simulink model "SimulinkAnalysisofCheetahTail"  (R2022a)
settings: Solver=ode4  StartTime=0.0  StopTime=1.5  FixedStep=0.001  RelTol=1e-3
undefined symbols (not defined in the file): B_cg_H, B_con_H, B_con_L, bar_len, cd_table, Cf, cl_table, g, gear_ratio, int_point_bar, int_point_tail, ITail, M_add, M_cg_H, M_cg_L, M_cg_W, Mb, Mm, Mt, psi3, rho, T_cg_H, T_fur_gap, T_length, T_width_major, T_width_minor, th2_initial, torque_constant, uncertainty_Forces, uncertainty_Position, Vf, windspeed
(part 17 of 21)

== matlab function SimulinkAnalysisofCheetahTail/Model/Forces/MATLAB Function1 ==
  data: int_point_tail input; A_output output; bar_len parameter; T_length parameter; T_width_major parameter
function A_output = fcn(int_point_tail, bar_len, T_length, T_width_major)

A_output = (T_length + bar_len-int_point_tail)/5*T_width_major;

== matlab function SimulinkAnalysisofCheetahTail/Model/Forces/CD_CL_tail_1/v_tail_1 ==
  data: v_tail_1_speed output; int_point_tail input; q input; dq input; B_con_H parameter; psi3 parameter; windspeed parameter; B_con_L parameter; M_cg_H parameter; M_cg_L parameter; M_cg_W parameter; T_fur_gap parameter; T_length parameter; bar_len parameter
function v_tail_1_speed = v_tail_1(int_point_tail,q,dq, B_con_H, psi3, windspeed, B_con_L, M_cg_H, M_cg_L, M_cg_W, T_fur_gap, T_length, bar_len)
%#codegen
[x,y,z,phi1,th1,psi1,phi2,th2] = deal(q(1),q(2),q(3),q(4),q(5),q(6),q(7),q(8));
[dx,dy,dz,dphi1,dth1,dpsi1,dphi2,dth2] = deal(dq(1),dq(2),dq(3),dq(4),dq(5),dq(6),dq(7),dq(8));
%    This function was generated by the Symbolic Math Toolbox version 9.0.
%    09-Feb-2022 11:07:13

t2 = cos(phi1);
t3 = cos(phi2);
t4 = cos(psi1);
t5 = cos(psi3);
t6 = cos(th1);
t7 = cos(th2);
t8 = sin(phi1);
t9 = sin(phi2);
t10 = sin(psi1);
t11 = sin(psi3);
t12 = sin(th1);
t13 = sin(th2);
t14 = M_cg_L+x;
t15 = M_cg_W+y;
t16 = M_cg_H+z;
t35 = T_length./1.0e+1;
t36 = bar_len./1.0e+1;
t37 = int_point_tail./1.0e+1;
t17 = B_con_L.*t6;
t18 = B_con_L.*t12;
t19 = t2.*t4;
t20 = t6.*t7;
t21 = t2.*t10;
t22 = t4.*t8;
t23 = t7.*t12;
t24 = t8.*t10;
t25 = t12.*t13;
t26 = B_con_H.*t2.*t6;
t28 = t6.*t14;
t29 = B_con_H.*t2.*t12;
t30 = B_con_H.*t6.*t8;
t33 = t12.*t14;
t40 = t6.*t9.*t13;
t42 = t6.*t10.*t13;
t44 = t8.*t9.*t12;
t47 = -t37;
t48 = t2.*t3.*t6;
t51 = t2.*t6.*t9;
t52 = t3.*t6.*t8;
t54 = t2.*t6.*t13;
t55 = t3.*t6.*t13;
t57 = t4.*t6.*t13;
t60 = t3.*t8.*t12;
t61 = t6.*t8.*t9;
t66 = t2.*t6.*t15;
t68 = t2.*t6.*t16;
t71 = t6.*t8.*t15;
t72 = t2.*t12.*t16;
t73 = t6.*t8.*t16;
t75 = t8.*t12.*t15;
t27 = t4.*t17;
t31 = t4.*t18;
t32 = t10.*t17;
t34 = t10.*t18;
t38 = t2.*t25;
t39 = t3.*t25;
t41 = t9.*t23;
t43 = t10.*t23;
t45 = t12.*t24;
t46 = t9.*t25;
t49 = t2.*t20;
t50 = t4.*t20;
t53 = t12.*t19;
t56 = t3.*t23;
t58 = t4.*t23;
t59 = t10.*t20;
t62 = t12.*t21;
t63 = t12.*t22;
t64 = B_con_H.*t6.*t19;
t65 = t4.*t28;
t67 = B_con_H.*t6.*t21;
t69 = t4.*t33;
t70 = t10.*t28;
t74 = t10.*t33;
t76 = -t29;
t77 = -t30;
t79 = -t44;
t84 = t3.*t6.*t22;
t85 = t13.*t48;
t88 = t3.*t8.*t20;
t89 = t6.*t13.*t19;
t90 = t4.*t55;
t93 = t3.*t6.*t24;
t94 = t6.*t9.*t22;
t95 = t2.*t40;
t97 = t8.*t9.*t20;
t98 = t6.*t13.*t21;
t100 = t3.*t42;
t101 = t4.*t40;
t103 = t6.*t9.*t24;
t107 = t10.*t40;
t109 = -t57;
t112 = t6.*t16.*t19;
t113 = t6.*t15.*t22;
t114 = t6.*t16.*t21;
t115 = t6.*t15.*t24;
t116 = -t66;
t117 = -t71;
t118 = -t72;
t119 = -t73;
t120 = t3.*t19.*t20;
t121 = t3.*t20.*t21;
t122 = t9.*t19.*t20;
t123 = t9.*t20.*t21;
t133 = t23+t54;
t194 = t35+t36+t47;
t78 = -t38;
t80 = -t45;
t81 = -t46;
t82 = t3.*t49;
t83 = t3.*t50;
t86 = t2.*t56;
t87 = t9.*t49;
t91 = t3.*t59;
t92 = t9.*t50;
t96 = t2.*t41;
t99 = t4.*t39;
t102 = t9.*t59;
t104 = -t49;
t105 = t10.*t39;
t106 = t4.*t46;
t108 = -t53;
t110 = -t59;
t111 = t10.*t46;
t125 = -t90;
t127 = -t97;
t131 = -t113;
t132 = -t115;
t134 = t21+t63;
t135 = t22+t62;
t136 = -t120;
t137 = -t121;
t144 = t5.*t133;
t148 = t11.*t133;
t152 = t51+t88;
t156 = t56+t85;
t157 = t58+t89;
t158 = t41+t95;
t159 = t43+t98;
t124 = -t82;
t126 = -t91;
t128 = -t102;
t129 = t4.*t81;
t130 = t10.*t81;
t138 = B_con_H.*t134;
t139 = B_con_H.*t135;
t140 = t20+t78;
t141 = t25+t104;
t142 = t19+t80;
t143 = t24+t108;
t145 = t3.*t134;
t146 = t3.*t135;
t147 = t7.*t135;
t149 = t9.*t134;
t150 = t9.*t135;
t151 = t13.*t135;
t160 = t15.*t134;
t161 = t15.*t135;
t162 = t16.*t134;
t163 = t16.*t135;
t173 = -t148;
t177 = t48+t127;
t178 = T_fur_gap.*t152;
t179 = T_fur_gap.*t156;
t180 = int_point_tail.*t152;
t181 = int_point_tail.*t156;
t202 = t40+t60+t96;
t205 = t55+t79+t86;
t206 = t52+t81+t87;
t229 = t94+t99+t136;
t231 = t103+t105+t137;
t239 = t152.*t194;
t240 = t156.*t194;
t153 = B_con_H.*t142;
t154 = B_con_H.*t143;
t155 = -t139;
t164 = t7.*t145;
t165 = t7.*t146;
t166 = t13.*t146;
t167 = t7.*t149;
t168 = t9.*t147;
t169 = t13.*t150;
t170 = t3.*t142;
t171 = t3.*t143;
t172 = t7.*t143;
t174 = t9.*t142;
t175 = t9.*t143;
t176 = t13.*t143;
t182 = t15.*t142;
t183 = t15.*t143;
t184 = -t161;
t185 = t16.*t142;
t186 = t16.*t143;
t187 = -t163;
t201 = t42+t147;
t203 = t110+t151;
t204 = t39+t61+t124;
t209 = T_fur_gap.*t205;
t210 = T_fur_gap.*t206;
t212 = int_point_tail.*t205;
t213 = int_point_tail.*t206;
t216 = -t5.*(t59-t151);
t218 = -t11.*(t59-t151);
t219 = t5.*t206;
t220 = t11.*t206;
t230 = t84+t122+t129;
t232 = t93+t123+t130;
t233 = T_fur_gap.*t229;
t234 = int_point_tail.*t229;
t235 = T_fur_gap.*t231;
t236 = int_point_tail.*t231;
t250 = t194.*t205;
t251 = t194.*t206;
t272 = t194.*t229;
t275 = t194.*t231;
t283 = t179+t181+t240;
t289 = t77+t116+t119+t178+t180+t239;
t188 = t7.*t170;
t189 = t7.*t171;
t190 = -t164;
t191 = t13.*t171;
t192 = t7.*t174;
t193 = t9.*t172;
t195 = t13.*t175;
t196 = -t170;
t197 = -t182;
t198 = -t183;
t207 = t50+t176;
t208 = T_fur_gap.*t204;
t211 = int_point_tail.*t204;
t214 = t109+t172;
t222 = t126+t166;
t224 = t128+t169;
t226 = -T_fur_gap.*(t91-t166);
t228 = -int_point_tail.*(t91-t166);
t238 = t167+t171;
t244 = -T_fur_gap.*(t164-t175);
t246 = -int_point_tail.*(t164-t175);
t247 = t144+t220;
t248 = t100+t165+t174;
t249 = t194.*t204;
t255 = t173+t219;
t268 = -t194.*(t91-t166);
t277 = -t194.*(t164-t175);
t288 = t210+t213+t251;
t293 = t17+t28+t75+t76+t118+t209+t212+t250;
t294 = t34+t67+t74+t114+t132+t235+t236+t275;
t295 = t31+t64+t69+t112+t131+t233+t234+t272;
t199 = -t188;
t200 = -t193;
t215 = t5.*t207;
t217 = t11.*t207;
t221 = t83+t191;
t223 = t92+t195;
t237 = t146+t192;
t242 = t175+t190;
t252 = T_fur_gap.*t248;
t253 = int_point_tail.*t248;
t254 = t125+t149+t189;
t257 = t107+t168+t196;
t278 = t194.*t248;
t291 = t226+t228+t268;
t292 = t18+t26+t33+t68+t117+t208+t211+t249;
t298 = t138+t162+t198+t244+t246+t277;
t225 = T_fur_gap.*t221;
t227 = int_point_tail.*t221;
t241 = t150+t199;
t256 = t101+t145+t200;
t258 = T_fur_gap.*t254;
t260 = int_point_tail.*t254;
t261 = T_fur_gap.*t257;
t263 = int_point_tail.*t257;
t265 = t194.*t221;
t266 = t5.*t257;
t269 = t11.*t257;
t279 = t194.*t254;
t281 = t194.*t257;
t300 = t32+t70+t155+t187+t197+t252+t253+t278;
t243 = T_fur_gap.*t241;
t245 = int_point_tail.*t241;
t259 = T_fur_gap.*t256;
t262 = int_point_tail.*t256;
t264 = t5.*t256;
t267 = t11.*t256;
t270 = -t258;
t271 = -t260;
t273 = -t266;
t276 = t194.*t241;
t280 = t194.*t256;
t282 = -t279;
t285 = t216+t269;
t290 = t225+t227+t265;
t297 = t261+t263+t281;
t274 = -t267;
t284 = t217+t264;
t287 = t218+t273;
t296 = t259+t262+t280;
t299 = t153+t184+t185+t243+t245+t276;
t301 = t27+t65+t154+t160+t186+t270+t271+t282;
t286 = t215+t274;
et1 = dphi1.*(t204.*(t30+t66+t73-t178-t180-t239)-t152.*t292+t241.*t300+t248.*t299+t301.*(t164-t175)-t254.*(-t138-t162+t183+T_fur_gap.*(t164-t175)+int_point_tail.*(t164-t175)+t194.*(t164-t175)))-dth2.*(t156.*t292+t204.*t283+t221.*t301-t254.*t290+t248.*(T_fur_gap.*(t91-t166)+int_point_tail.*(t91-t166)+t194.*(t91-t166))+t300.*(t91-t166))+dy.*(t134.*t254+t142.*t248+t6.*t8.*t204)+dz.*(t135.*t248+t143.*t254-t2.*t6.*t204)-dphi2.*(t204.*t288+t206.*t292-t248.*t297+t254.*t296-t256.*t301-t257.*t300);
et2 = -dth1.*(t204.*t293+t205.*t292-t229.*t301-t231.*t300-t248.*t294+t254.*t295)-dx.*(t12.*t204-t4.*t6.*t254+t6.*t10.*t248)+t5.*t248.*windspeed-t11.*t254.*windspeed;
et3 = dphi2.*(t297.*(t269-t5.*(t59-t151))+t247.*t288-t286.*t296-t11.*t204.*t292-t11.*t248.*t300+t11.*t254.*t301)+dth1.*(t294.*(t269-t5.*(t59-t151))+t247.*t293-t286.*t295+t292.*(t5.*t140-t11.*t202)-t301.*(t5.*t157+t11.*t230)-t300.*(t5.*t159+t11.*t232))+dy.*(t142.*(t269-t5.*(t59-t151))+t134.*t286-t6.*t8.*t247)+dz.*(t135.*(t269-t5.*(t59-t151))+t143.*t286+t2.*t6.*t247);
et4 = -dth2.*(-t247.*t283-t286.*t290+(t269-t5.*(t59-t151)).*(T_fur_gap.*(t91-t166)+int_point_tail.*(t91-t166)+t194.*(t91-t166))+t292.*(t5.*t141+t11.*t158)+t301.*(t11.*t223+t5.*(t57-t172))+t300.*(t5.*t201+t11.*(t102-t169)))+dx.*(t12.*t247-t6.*t10.*(t269-t5.*(t59-t151))+t4.*t6.*t286);
et5 = -dphi1.*(t247.*(t30+t66+t73-t178-t180-t239)-t299.*(t269-t5.*(t59-t151))-t301.*(t11.*t238+t5.*t13.*t134)+t300.*(t11.*t237+t5.*t13.*t142)+t286.*(-t138-t162+t183+T_fur_gap.*(t164-t175)+int_point_tail.*(t164-t175)+t194.*(t164-t175))-t292.*(t11.*t177-t5.*t6.*t8.*t13))+t5.*windspeed.*(t269-t5.*(t59-t151))-t11.*t286.*windspeed;
et6 = -dphi1.*(t299.*(t266+t11.*(t59-t151))+t301.*(t5.*t238-t11.*t13.*t134)-t300.*(t5.*t237-t11.*t13.*t142)+(t148-t219).*(t30+t66+t73-t178-t180-t239)+t284.*(-t138-t162+t183+T_fur_gap.*(t164-t175)+int_point_tail.*(t164-t175)+t194.*(t164-t175))+t292.*(t5.*t177+t6.*t8.*t11.*t13))-dphi2.*(t297.*(t266+t11.*(t59-t151))+t284.*t296-t288.*(t148-t219)-t5.*t204.*t292-t5.*t248.*t300+t5.*t254.*t301);
et7 = -dth1.*(t294.*(t266+t11.*(t59-t151))+t284.*t295-t293.*(t148-t219)-t292.*(t11.*t140+t5.*t202)+t301.*(t11.*t157-t5.*t230)+t300.*(t11.*t159-t5.*t232))-dy.*(t142.*(t266+t11.*(t59-t151))-t134.*t284+t6.*t8.*(t148-t219))+dz.*(-t135.*(t266+t11.*(t59-t151))+t143.*t284+t2.*t6.*(t148-t219));
et8 = dth2.*(t284.*t290+(t266+t11.*(t59-t151)).*(T_fur_gap.*(t91-t166)+int_point_tail.*(t91-t166)+t194.*(t91-t166))+t283.*(t148-t219)-t292.*(t11.*t141-t5.*t158)+t301.*(t5.*t223-t11.*(t57-t172))-t300.*(t11.*t201-t5.*(t102-t169)))+dx.*(t12.*(t148-t219)+t6.*t10.*(t266+t11.*(t59-t151))+t4.*t6.*t284)-t5.*windspeed.*(t266+t11.*(t59-t151))-t11.*t284.*windspeed;
v_tail_1_speed = sqrt(abs(et3+et4+et5).^2+abs(et6+et7+et8).^2+abs(et1+et2).^2);

== matlab function SimulinkAnalysisofCheetahTail/Model/Forces/CD_CL_tail_1/aoa_tail_1 ==
  data: int_point_tail input; q input; dq input; aoa_tail_1 output; psi3 parameter; windspeed parameter; B_con_H parameter; B_con_L parameter; M_cg_H parameter; M_cg_L parameter; M_cg_W parameter; T_fur_gap parameter; T_length parameter; bar_len parameter
function aoa_tail_1 = aoa_tail_1(int_point_tail,q,dq, psi3, windspeed, B_con_H, B_con_L, M_cg_H, M_cg_L, M_cg_W, T_fur_gap, T_length, bar_len)
%#codegen
[x,y,z,phi1,th1,psi1,phi2,th2] = deal(q(1),q(2),q(3),q(4),q(5),q(6),q(7),q(8));
[dx,dy,dz,dphi1,dth1,dpsi1,dphi2,dth2] = deal(dq(1),dq(2),dq(3),dq(4),dq(5),dq(6),dq(7),dq(8));
%    This function was generated by the Symbolic Math Toolbox version 9.0.
%    09-Feb-2022 11:07:17

t2 = cos(phi1);
t3 = cos(phi2);
t4 = cos(psi1);
t5 = cos(psi3);
t6 = cos(th1);
t7 = cos(th2);
t8 = sin(phi1);
t9 = sin(phi2);
t10 = sin(psi1);
t11 = sin(psi3);
t12 = sin(th1);
t13 = sin(th2);
t14 = M_cg_L+x;
t15 = M_cg_W+y;
t16 = M_cg_H+z;
t33 = T_length./1.0e+1;
t34 = bar_len./1.0e+1;
t35 = int_point_tail./1.0e+1;
t17 = B_con_L.*t6;
t18 = B_con_L.*t12;
t19 = t2.*t4;
t20 = t2.*t10;
t21 = t4.*t8;
t22 = t7.*t12;
t23 = t8.*t10;
t24 = B_con_H.*t2.*t6;
t26 = t6.*t14;
t27 = B_con_H.*t2.*t12;
t28 = B_con_H.*t6.*t8;
t31 = t12.*t14;
t36 = t3.*t12.*t13;
t37 = t8.*t9.*t12;
t39 = t9.*t12.*t13;
t40 = -t35;
t41 = t4.*t6.*t7;
t42 = t2.*t6.*t9;
t43 = t3.*t6.*t8;
t45 = t2.*t6.*t13;
t46 = t3.*t6.*t13;
t48 = t6.*t7.*t10;
t49 = t6.*t8.*t9;
t54 = t2.*t6.*t15;
t56 = t2.*t6.*t16;
t59 = t6.*t8.*t15;
t60 = t2.*t12.*t16;
t61 = t6.*t8.*t16;
t63 = t8.*t12.*t15;
t69 = t2.*t3.*t6.*t7;
t80 = t4.*t6.*t9.*t13;
t83 = t6.*t9.*t10.*t13;
t25 = t4.*t17;
t29 = t4.*t18;
t30 = t10.*t17;
t32 = t10.*t18;
t38 = t12.*t23;
t44 = t12.*t19;
t47 = t3.*t22;
t50 = t12.*t20;
t51 = t12.*t21;
t52 = B_con_H.*t6.*t19;
t53 = t4.*t26;
t55 = B_con_H.*t6.*t20;
t57 = t4.*t31;
t58 = t10.*t26;
t62 = t10.*t31;
t64 = -t27;
t65 = -t28;
t66 = -t37;
t68 = -t39;
t70 = t3.*t41;
t71 = t3.*t45;
t73 = t7.*t42;
t74 = t7.*t43;
t75 = t4.*t46;
t76 = t3.*t48;
t77 = t6.*t9.*t21;
t78 = t4.*t36;
t79 = t10.*t46;
t81 = t6.*t9.*t23;
t82 = t10.*t36;
t85 = -t48;
t86 = t6.*t16.*t19;
t87 = t6.*t15.*t21;
t88 = t6.*t16.*t20;
t89 = t6.*t15.*t23;
t90 = -t54;
t91 = -t59;
t92 = -t60;
t93 = -t61;
t94 = t3.*t6.*t7.*t19;
t95 = t3.*t6.*t7.*t20;
t96 = -t69;
t101 = t22+t45;
t148 = t33+t34+t40;
t67 = -t38;
t72 = t2.*t47;
t84 = -t44;
t97 = -t75;
t98 = -t76;
t99 = -t87;
t100 = -t89;
t102 = t20+t51;
t103 = t21+t50;
t104 = -t94;
t105 = -t95;
t111 = t11.*t101;
t115 = t42+t74;
t119 = t47+t71;
t155 = t36+t49+t96;
t157 = t43+t68+t73;
t106 = B_con_H.*t102;
t107 = B_con_H.*t103;
t108 = t19+t67;
t109 = t23+t84;
t110 = t3.*t102;
t112 = t9.*t102;
t113 = t9.*t103;
t114 = t13.*t103;
t120 = t15.*t102;
t121 = t15.*t103;
t122 = t16.*t102;
t123 = t16.*t103;
t125 = t3.*t7.*t103;
t129 = -t111;
t133 = T_fur_gap.*t115;
t134 = T_fur_gap.*t119;
t135 = int_point_tail.*t115;
t136 = int_point_tail.*t119;
t156 = t46+t66+t72;
t159 = T_fur_gap.*t155;
t161 = T_fur_gap.*t157;
t162 = int_point_tail.*t155;
t164 = int_point_tail.*t157;
t167 = t5.*t157;
t174 = t77+t78+t104;
t175 = t81+t82+t105;
t180 = t115.*t148;
t181 = t119.*t148;
t189 = t148.*t155;
t191 = t148.*t157;
t116 = B_con_H.*t108;
t117 = B_con_H.*t109;
t118 = -t107;
t124 = t7.*t110;
t126 = t3.*t114;
t127 = t7.*t113;
t128 = t3.*t108;
t130 = t9.*t108;
t131 = t9.*t109;
t132 = t13.*t109;
t137 = t15.*t108;
t138 = t15.*t109;
t139 = -t121;
t140 = t16.*t108;
t141 = t16.*t109;
t142 = -t123;
t144 = t3.*t7.*t109;
t154 = t85+t114;
t160 = T_fur_gap.*t156;
t163 = int_point_tail.*t156;
t166 = -t11.*(t48-t114);
t176 = T_fur_gap.*t174;
t177 = int_point_tail.*t174;
t178 = T_fur_gap.*t175;
t179 = int_point_tail.*t175;
t190 = t148.*t156;
t195 = t129+t167;
t210 = t148.*t174;
t212 = t148.*t175;
t220 = t134+t136+t181;
t223 = t161+t164+t191;
t224 = t65+t90+t93+t133+t135+t180;
t227 = t18+t24+t31+t56+t91+t159+t162+t189;
t143 = t7.*t128;
t145 = -t124;
t146 = t3.*t132;
t147 = t7.*t131;
t149 = -t128;
t150 = -t137;
t151 = -t138;
t158 = t41+t132;
t169 = t98+t126;
t171 = -T_fur_gap.*(t76-t126);
t173 = -int_point_tail.*(t76-t126);
t185 = -T_fur_gap.*(t124-t131);
t187 = -int_point_tail.*(t124-t131);
t188 = t79+t125+t130;
t194 = t97+t112+t144;
t207 = -t148.*(t76-t126);
t214 = -t148.*(t124-t131);
t228 = t17+t26+t63+t64+t92+t160+t163+t190;
t229 = t32+t55+t62+t88+t100+t178+t179+t212;
t230 = t29+t52+t57+t86+t99+t176+t177+t210;
t152 = -t143;
t153 = -t147;
t165 = t11.*t158;
t168 = t70+t146;
t183 = t131+t145;
t192 = T_fur_gap.*t188;
t193 = int_point_tail.*t188;
t197 = t83+t127+t149;
t198 = T_fur_gap.*t194;
t200 = int_point_tail.*t194;
t215 = t148.*t188;
t216 = t148.*t194;
t226 = t171+t173+t207;
t233 = t106+t122+t151+t185+t187+t214;
t170 = T_fur_gap.*t168;
t172 = int_point_tail.*t168;
t182 = t113+t152;
t196 = t80+t110+t153;
t201 = T_fur_gap.*t197;
t203 = int_point_tail.*t197;
t205 = t148.*t168;
t206 = t5.*t197;
t208 = -t198;
t209 = -t200;
t218 = t148.*t197;
t219 = -t216;
t235 = t30+t58+t118+t142+t150+t192+t193+t215;
t184 = T_fur_gap.*t182;
t186 = int_point_tail.*t182;
t199 = T_fur_gap.*t196;
t202 = int_point_tail.*t196;
t204 = t5.*t196;
t211 = -t206;
t213 = t148.*t182;
t217 = t148.*t196;
t225 = t170+t172+t205;
t232 = t201+t203+t218;
t236 = t25+t53+t117+t120+t141+t208+t209+t219;
t221 = t165+t204;
t222 = t166+t211;
t231 = t199+t202+t217;
t234 = t116+t139+t140+t184+t186+t213;
et1 = dphi1.*(t234.*(t206+t11.*(t48-t114))+(t111-t167).*(t28+t54+t61-t133-t135-t180)+t221.*(-t106-t122+t138+T_fur_gap.*(t124-t131)+int_point_tail.*(t124-t131)+t148.*(t124-t131))-t227.*(t5.*(t7.*t49-t2.*t3.*t6)-t6.*t8.*t11.*t13)+t236.*(t5.*(t3.*t109+t7.*t112)-t11.*t13.*t102)-t235.*(t5.*(t3.*t103+t7.*t130)-t11.*t13.*t108))+dphi2.*(t232.*(t206+t11.*(t48-t114))+t221.*t231-t223.*(t111-t167)-t5.*t155.*t227-t5.*t188.*t235+t5.*t194.*t236);
et2 = dth1.*(t229.*(t206+t11.*(t48-t114))+t221.*t230-t228.*(t111-t167)-t227.*(t11.*(t6.*t7-t2.*t12.*t13)+t5.*(t3.*t8.*t12+t6.*t9.*t13+t2.*t9.*t22))+t236.*(t11.*(t4.*t22+t6.*t13.*t19)-t5.*(t4.*t68+t3.*t6.*t21+t6.*t7.*t9.*t19))+t235.*(t11.*(t10.*t22+t6.*t13.*t20)-t5.*(t10.*t68+t3.*t6.*t23+t6.*t7.*t9.*t20)))+dy.*(t108.*(t206+t11.*(t48-t114))-t102.*t221+t6.*t8.*(t111-t167))-dz.*(-t103.*(t206+t11.*(t48-t114))+t109.*t221+t2.*t6.*(t111-t167));
et3 = -dth2.*(-t227.*(t11.*(t12.*t13-t2.*t6.*t7)-t5.*(t9.*t22+t13.*t42))-t235.*(t11.*(t7.*t103+t6.*t10.*t13)-t5.*(t9.*t48-t13.*t113))+t236.*(t11.*(t7.*t109-t4.*t6.*t13)+t5.*(t9.*t41+t13.*t131))+t221.*t225+(t206+t11.*(t48-t114)).*(T_fur_gap.*(t76-t126)+int_point_tail.*(t76-t126)+t148.*(t76-t126))+t220.*(t111-t167))-dx.*(t12.*(t111-t167)+t6.*t10.*(t206+t11.*(t48-t114))+t4.*t6.*t221)+t5.*windspeed.*(t206+t11.*(t48-t114))+t11.*t221.*windspeed;
et4 = -dphi1.*(t155.*(t28+t54+t61-t133-t135-t180)-t115.*t227+t182.*t235+t188.*t234+t236.*(t124-t131)-t194.*(-t106-t122+t138+T_fur_gap.*(t124-t131)+int_point_tail.*(t124-t131)+t148.*(t124-t131)))+dth2.*(t119.*t227+t155.*t220+t168.*t236-t194.*t225+t188.*(T_fur_gap.*(t76-t126)+int_point_tail.*(t76-t126)+t148.*(t76-t126))+t235.*(t76-t126))-dy.*(t102.*t194+t108.*t188+t6.*t8.*t155)-dz.*(t103.*t188+t109.*t194-t2.*t6.*t155)+dphi2.*(t155.*t223+t157.*t227-t188.*t232+t194.*t231-t196.*t236-t197.*t235);
et5 = dth1.*(t155.*t228+t156.*t227-t174.*t236-t175.*t235-t188.*t229+t194.*t230)+dx.*(t12.*t155-t4.*t6.*t194+t6.*t10.*t188)-t5.*t188.*windspeed+t11.*t194.*windspeed;
aoa_tail_1 = th2-atan((et4+et5)./(et1+et2+et3));

== matlab function SimulinkAnalysisofCheetahTail/Model/Forces/CD_CL_tail_2/v_tail_2 ==
  data: int_point_tail input; q input; dq input; v_tail_2_speed output; psi3 parameter; windspeed parameter; B_con_H parameter; B_con_L parameter; M_cg_H parameter; M_cg_L parameter; M_cg_W parameter; T_fur_gap parameter; T_length parameter; bar_len parameter
function v_tail_2_speed = v_tail_2(int_point_tail,q,dq, psi3, windspeed, B_con_H, B_con_L, M_cg_H, M_cg_L, M_cg_W, T_fur_gap, T_length, bar_len)
%#codegen
[x,y,z,phi1,th1,psi1,phi2,th2] = deal(q(1),q(2),q(3),q(4),q(5),q(6),q(7),q(8));
[dx,dy,dz,dphi1,dth1,dpsi1,dphi2,dth2] = deal(dq(1),dq(2),dq(3),dq(4),dq(5),dq(6),dq(7),dq(8));
%    This function was generated by the Symbolic Math Toolbox version 9.0.
%    09-Feb-2022 11:07:20

t2 = cos(phi1);
t3 = cos(phi2);
t4 = cos(psi1);
t5 = cos(psi3);
t6 = cos(th1);
t7 = cos(th2);
t8 = sin(phi1);
t9 = sin(phi2);
t10 = sin(psi1);
t11 = sin(psi3);
t12 = sin(th1);
t13 = sin(th2);
t14 = M_cg_L+x;
t15 = M_cg_W+y;
t16 = M_cg_H+z;
t35 = T_length.*(3.0./1.0e+1);
t36 = bar_len.*(3.0./1.0e+1);
t37 = int_point_tail.*(3.0./1.0e+1);
t17 = B_con_L.*t6;
t18 = B_con_L.*t12;
t19 = t2.*t4;
t20 = t6.*t7;
t21 = t2.*t10;
t22 = t4.*t8;
t23 = t7.*t12;
t24 = t8.*t10;
t25 = t12.*t13;
t26 = B_con_H.*t2.*t6;
t28 = t6.*t14;
t29 = B_con_H.*t2.*t12;
t30 = B_con_H.*t6.*t8;
t33 = t12.*t14;
t40 = t6.*t9.*t13;
t42 = t6.*t10.*t13;
t44 = t8.*t9.*t12;
t47 = -t37;
t48 = t2.*t3.*t6;
t51 = t2.*t6.*t9;
t52 = t3.*t6.*t8;
t54 = t2.*t6.*t13;
t55 = t3.*t6.*t13;
t57 = t4.*t6.*t13;
t60 = t3.*t8.*t12;
t61 = t6.*t8.*t9;
t66 = t2.*t6.*t15;
t68 = t2.*t6.*t16;
t71 = t6.*t8.*t15;
t72 = t2.*t12.*t16;
t73 = t6.*t8.*t16;
t75 = t8.*t12.*t15;
t27 = t4.*t17;
t31 = t4.*t18;
t32 = t10.*t17;
t34 = t10.*t18;
t38 = t2.*t25;
t39 = t3.*t25;
t41 = t9.*t23;
t43 = t10.*t23;
t45 = t12.*t24;
t46 = t9.*t25;
t49 = t2.*t20;
t50 = t4.*t20;
t53 = t12.*t19;
t56 = t3.*t23;
t58 = t4.*t23;
t59 = t10.*t20;
t62 = t12.*t21;
t63 = t12.*t22;
t64 = B_con_H.*t6.*t19;
t65 = t4.*t28;
t67 = B_con_H.*t6.*t21;
t69 = t4.*t33;
t70 = t10.*t28;
t74 = t10.*t33;
t76 = -t29;
t77 = -t30;
t79 = -t44;
t84 = t3.*t6.*t22;
t85 = t13.*t48;
t88 = t3.*t8.*t20;
t89 = t6.*t13.*t19;
t90 = t4.*t55;
t93 = t3.*t6.*t24;
t94 = t6.*t9.*t22;
t95 = t2.*t40;
t97 = t8.*t9.*t20;
t98 = t6.*t13.*t21;
t100 = t3.*t42;
t101 = t4.*t40;
t103 = t6.*t9.*t24;
t107 = t10.*t40;
t109 = -t57;
t112 = t6.*t16.*t19;
t113 = t6.*t15.*t22;
t114 = t6.*t16.*t21;
t115 = t6.*t15.*t24;
t116 = -t66;
t117 = -t71;
t118 = -t72;
t119 = -t73;
t120 = t3.*t19.*t20;
t121 = t3.*t20.*t21;
t122 = t9.*t19.*t20;
t123 = t9.*t20.*t21;
t133 = t23+t54;
t194 = t35+t36+t47;
t78 = -t38;
t80 = -t45;
t81 = -t46;
t82 = t3.*t49;
t83 = t3.*t50;
t86 = t2.*t56;
t87 = t9.*t49;
t91 = t3.*t59;
t92 = t9.*t50;
t96 = t2.*t41;
t99 = t4.*t39;
t102 = t9.*t59;
t104 = -t49;
t105 = t10.*t39;
t106 = t4.*t46;
t108 = -t53;
t110 = -t59;
t111 = t10.*t46;
t125 = -t90;
t127 = -t97;
t131 = -t113;
t132 = -t115;
t134 = t21+t63;
t135 = t22+t62;
t136 = -t120;
t137 = -t121;
t144 = t5.*t133;
t148 = t11.*t133;
t152 = t51+t88;
t156 = t56+t85;
t157 = t58+t89;
t158 = t41+t95;
t159 = t43+t98;
t124 = -t82;
t126 = -t91;
t128 = -t102;
t129 = t4.*t81;
t130 = t10.*t81;
t138 = B_con_H.*t134;
t139 = B_con_H.*t135;
t140 = t20+t78;
t141 = t25+t104;
t142 = t19+t80;
t143 = t24+t108;
t145 = t3.*t134;
t146 = t3.*t135;
t147 = t7.*t135;
t149 = t9.*t134;
t150 = t9.*t135;
t151 = t13.*t135;
t160 = t15.*t134;
t161 = t15.*t135;
t162 = t16.*t134;
t163 = t16.*t135;
t173 = -t148;
t177 = t48+t127;
t178 = T_fur_gap.*t152;
t179 = T_fur_gap.*t156;
t180 = int_point_tail.*t152;
t181 = int_point_tail.*t156;
t202 = t40+t60+t96;
t205 = t55+t79+t86;
t206 = t52+t81+t87;
t229 = t94+t99+t136;
t231 = t103+t105+t137;
t239 = t152.*t194;
t240 = t156.*t194;
t153 = B_con_H.*t142;
t154 = B_con_H.*t143;
t155 = -t139;
t164 = t7.*t145;
t165 = t7.*t146;
t166 = t13.*t146;
t167 = t7.*t149;
t168 = t9.*t147;
t169 = t13.*t150;
t170 = t3.*t142;
t171 = t3.*t143;
t172 = t7.*t143;
t174 = t9.*t142;
t175 = t9.*t143;
t176 = t13.*t143;
t182 = t15.*t142;
t183 = t15.*t143;
t184 = -t161;
t185 = t16.*t142;
t186 = t16.*t143;
t187 = -t163;
t201 = t42+t147;
t203 = t110+t151;
t204 = t39+t61+t124;
t209 = T_fur_gap.*t205;
t210 = T_fur_gap.*t206;
t212 = int_point_tail.*t205;
t213 = int_point_tail.*t206;
t216 = -t5.*(t59-t151);
t218 = -t11.*(t59-t151);
t219 = t5.*t206;
t220 = t11.*t206;
t230 = t84+t122+t129;
t232 = t93+t123+t130;
t233 = T_fur_gap.*t229;
t234 = int_point_tail.*t229;
t235 = T_fur_gap.*t231;
t236 = int_point_tail.*t231;
t250 = t194.*t205;
t251 = t194.*t206;
t272 = t194.*t229;
t275 = t194.*t231;
t283 = t179+t181+t240;
t289 = t77+t116+t119+t178+t180+t239;
t188 = t7.*t170;
t189 = t7.*t171;
t190 = -t164;
t191 = t13.*t171;
t192 = t7.*t174;
t193 = t9.*t172;
t195 = t13.*t175;
t196 = -t170;
t197 = -t182;
t198 = -t183;
t207 = t50+t176;
t208 = T_fur_gap.*t204;
t211 = int_point_tail.*t204;
t214 = t109+t172;
t222 = t126+t166;
t224 = t128+t169;
t226 = -T_fur_gap.*(t91-t166);
t228 = -int_point_tail.*(t91-t166);
t238 = t167+t171;
t244 = -T_fur_gap.*(t164-t175);
t246 = -int_point_tail.*(t164-t175);
t247 = t144+t220;
t248 = t100+t165+t174;
t249 = t194.*t204;
t255 = t173+t219;
t268 = -t194.*(t91-t166);
t277 = -t194.*(t164-t175);
t288 = t210+t213+t251;
t293 = t17+t28+t75+t76+t118+t209+t212+t250;
t294 = t34+t67+t74+t114+t132+t235+t236+t275;
t295 = t31+t64+t69+t112+t131+t233+t234+t272;
t199 = -t188;
t200 = -t193;
t215 = t5.*t207;
t217 = t11.*t207;
t221 = t83+t191;
t223 = t92+t195;
t237 = t146+t192;
t242 = t175+t190;
t252 = T_fur_gap.*t248;
t253 = int_point_tail.*t248;
t254 = t125+t149+t189;
t257 = t107+t168+t196;
t278 = t194.*t248;
t291 = t226+t228+t268;
t292 = t18+t26+t33+t68+t117+t208+t211+t249;
t298 = t138+t162+t198+t244+t246+t277;
t225 = T_fur_gap.*t221;
t227 = int_point_tail.*t221;
t241 = t150+t199;
t256 = t101+t145+t200;
t258 = T_fur_gap.*t254;
t260 = int_point_tail.*t254;
t261 = T_fur_gap.*t257;
t263 = int_point_tail.*t257;
t265 = t194.*t221;
t266 = t5.*t257;
t269 = t11.*t257;
t279 = t194.*t254;
t281 = t194.*t257;
t300 = t32+t70+t155+t187+t197+t252+t253+t278;
t243 = T_fur_gap.*t241;
t245 = int_point_tail.*t241;
t259 = T_fur_gap.*t256;
t262 = int_point_tail.*t256;
t264 = t5.*t256;
t267 = t11.*t256;
t270 = -t258;
t271 = -t260;
t273 = -t266;
t276 = t194.*t241;
t280 = t194.*t256;
t282 = -t279;
t285 = t216+t269;
t290 = t225+t227+t265;
t297 = t261+t263+t281;
t274 = -t267;
t284 = t217+t264;
t287 = t218+t273;
t296 = t259+t262+t280;
t299 = t153+t184+t185+t243+t245+t276;
t301 = t27+t65+t154+t160+t186+t270+t271+t282;
t286 = t215+t274;
et1 = dphi1.*(t204.*(t30+t66+t73-t178-t180-t239)-t152.*t292+t241.*t300+t248.*t299+t301.*(t164-t175)-t254.*(-t138-t162+t183+T_fur_gap.*(t164-t175)+int_point_tail.*(t164-t175)+t194.*(t164-t175)))-dth2.*(t156.*t292+t204.*t283+t221.*t301-t254.*t290+t248.*(T_fur_gap.*(t91-t166)+int_point_tail.*(t91-t166)+t194.*(t91-t166))+t300.*(t91-t166))+dy.*(t134.*t254+t142.*t248+t6.*t8.*t204)+dz.*(t135.*t248+t143.*t254-t2.*t6.*t204)-dphi2.*(t204.*t288+t206.*t292-t248.*t297+t254.*t296-t256.*t301-t257.*t300);
et2 = -dth1.*(t204.*t293+t205.*t292-t229.*t301-t231.*t300-t248.*t294+t254.*t295)-dx.*(t12.*t204-t4.*t6.*t254+t6.*t10.*t248)+t5.*t248.*windspeed-t11.*t254.*windspeed;
et3 = dphi2.*(t297.*(t269-t5.*(t59-t151))+t247.*t288-t286.*t296-t11.*t204.*t292-t11.*t248.*t300+t11.*t254.*t301)+dth1.*(t294.*(t269-t5.*(t59-t151))+t247.*t293-t286.*t295+t292.*(t5.*t140-t11.*t202)-t301.*(t5.*t157+t11.*t230)-t300.*(t5.*t159+t11.*t232))+dy.*(t142.*(t269-t5.*(t59-t151))+t134.*t286-t6.*t8.*t247)+dz.*(t135.*(t269-t5.*(t59-t151))+t143.*t286+t2.*t6.*t247);
et4 = -dth2.*(-t247.*t283-t286.*t290+(t269-t5.*(t59-t151)).*(T_fur_gap.*(t91-t166)+int_point_tail.*(t91-t166)+t194.*(t91-t166))+t292.*(t5.*t141+t11.*t158)+t301.*(t11.*t223+t5.*(t57-t172))+t300.*(t5.*t201+t11.*(t102-t169)))+dx.*(t12.*t247-t6.*t10.*(t269-t5.*(t59-t151))+t4.*t6.*t286);
et5 = -dphi1.*(t247.*(t30+t66+t73-t178-t180-t239)-t299.*(t269-t5.*(t59-t151))-t301.*(t11.*t238+t5.*t13.*t134)+t300.*(t11.*t237+t5.*t13.*t142)+t286.*(-t138-t162+t183+T_fur_gap.*(t164-t175)+int_point_tail.*(t164-t175)+t194.*(t164-t175))-t292.*(t11.*t177-t5.*t6.*t8.*t13))+t5.*windspeed.*(t269-t5.*(t59-t151))-t11.*t286.*windspeed;
et6 = -dphi1.*(t299.*(t266+t11.*(t59-t151))+t301.*(t5.*t238-t11.*t13.*t134)-t300.*(t5.*t237-t11.*t13.*t142)+(t148-t219).*(t30+t66+t73-t178-t180-t239)+t284.*(-t138-t162+t183+T_fur_gap.*(t164-t175)+int_point_tail.*(t164-t175)+t194.*(t164-t175))+t292.*(t5.*t177+t6.*t8.*t11.*t13))-dphi2.*(t297.*(t266+t11.*(t59-t151))+t284.*t296-t288.*(t148-t219)-t5.*t204.*t292-t5.*t248.*t300+t5.*t254.*t301);
et7 = -dth1.*(t294.*(t266+t11.*(t59-t151))+t284.*t295-t293.*(t148-t219)-t292.*(t11.*t140+t5.*t202)+t301.*(t11.*t157-t5.*t230)+t300.*(t11.*t159-t5.*t232))-dy.*(t142.*(t266+t11.*(t59-t151))-t134.*t284+t6.*t8.*(t148-t219))+dz.*(-t135.*(t266+t11.*(t59-t151))+t143.*t284+t2.*t6.*(t148-t219));
et8 = dth2.*(t284.*t290+(t266+t11.*(t59-t151)).*(T_fur_gap.*(t91-t166)+int_point_tail.*(t91-t166)+t194.*(t91-t166))+t283.*(t148-t219)-t292.*(t11.*t141-t5.*t158)+t301.*(t5.*t223-t11.*(t57-t172))-t300.*(t11.*t201-t5.*(t102-t169)))+dx.*(t12.*(t148-t219)+t6.*t10.*(t266+t11.*(t59-t151))+t4.*t6.*t284)-t5.*windspeed.*(t266+t11.*(t59-t151))-t11.*t284.*windspeed;
v_tail_2_speed = sqrt(abs(et3+et4+et5).^2+abs(et6+et7+et8).^2+abs(et1+et2).^2);

== matlab function SimulinkAnalysisofCheetahTail/Model/Forces/CD_CL_tail_2/aoa_tail_2 ==
  data: int_point_tail input; q input; dq input; aoa_tail_2 output; psi3 parameter; windspeed parameter; B_con_H parameter; B_con_L parameter; M_cg_H parameter; M_cg_L parameter; M_cg_W parameter; T_fur_gap parameter; T_length parameter; bar_len parameter
function aoa_tail_2 = aoa_tail_2(int_point_tail,q,dq, psi3, windspeed, B_con_H, B_con_L, M_cg_H, M_cg_L, M_cg_W, T_fur_gap, T_length, bar_len)
%#codegen
[x,y,z,phi1,th1,psi1,phi2,th2] = deal(q(1),q(2),q(3),q(4),q(5),q(6),q(7),q(8));
[dx,dy,dz,dphi1,dth1,dpsi1,dphi2,dth2] = deal(dq(1),dq(2),dq(3),dq(4),dq(5),dq(6),dq(7),dq(8));
%    This function was generated by the Symbolic Math Toolbox version 9.0.
%    09-Feb-2022 11:07:23

t2 = cos(phi1);
t3 = cos(phi2);
t4 = cos(psi1);
t5 = cos(psi3);
t6 = cos(th1);
t7 = cos(th2);
t8 = sin(phi1);
t9 = sin(phi2);
t10 = sin(psi1);
t11 = sin(psi3);
t12 = sin(th1);
t13 = sin(th2);
t14 = M_cg_L+x;
t15 = M_cg_W+y;
t16 = M_cg_H+z;
t33 = T_length.*(3.0./1.0e+1);
t34 = bar_len.*(3.0./1.0e+1);
t35 = int_point_tail.*(3.0./1.0e+1);
t17 = B_con_L.*t6;
t18 = B_con_L.*t12;
t19 = t2.*t4;
t20 = t2.*t10;
t21 = t4.*t8;
t22 = t7.*t12;
t23 = t8.*t10;
t24 = B_con_H.*t2.*t6;
t26 = t6.*t14;
t27 = B_con_H.*t2.*t12;
t28 = B_con_H.*t6.*t8;
t31 = t12.*t14;
t36 = t3.*t12.*t13;
t37 = t8.*t9.*t12;
t39 = t9.*t12.*t13;
t40 = -t35;
t41 = t4.*t6.*t7;
t42 = t2.*t6.*t9;
t43 = t3.*t6.*t8;
t45 = t2.*t6.*t13;
t46 = t3.*t6.*t13;
t48 = t6.*t7.*t10;
t49 = t6.*t8.*t9;
t54 = t2.*t6.*t15;
t56 = t2.*t6.*t16;
t59 = t6.*t8.*t15;
t60 = t2.*t12.*t16;
t61 = t6.*t8.*t16;
t63 = t8.*t12.*t15;
t69 = t2.*t3.*t6.*t7;
t80 = t4.*t6.*t9.*t13;
t83 = t6.*t9.*t10.*t13;
t25 = t4.*t17;
t29 = t4.*t18;
t30 = t10.*t17;
t32 = t10.*t18;
t38 = t12.*t23;
t44 = t12.*t19;
t47 = t3.*t22;
t50 = t12.*t20;
t51 = t12.*t21;
t52 = B_con_H.*t6.*t19;
t53 = t4.*t26;
t55 = B_con_H.*t6.*t20;
t57 = t4.*t31;
t58 = t10.*t26;
t62 = t10.*t31;
t64 = -t27;
t65 = -t28;
t66 = -t37;
t68 = -t39;
t70 = t3.*t41;
t71 = t3.*t45;
t73 = t7.*t42;
t74 = t7.*t43;
t75 = t4.*t46;
t76 = t3.*t48;
t77 = t6.*t9.*t21;
t78 = t4.*t36;
t79 = t10.*t46;
t81 = t6.*t9.*t23;
t82 = t10.*t36;
t85 = -t48;
t86 = t6.*t16.*t19;
t87 = t6.*t15.*t21;
t88 = t6.*t16.*t20;
t89 = t6.*t15.*t23;
t90 = -t54;
t91 = -t59;
t92 = -t60;
t93 = -t61;
t94 = t3.*t6.*t7.*t19;
t95 = t3.*t6.*t7.*t20;
t96 = -t69;
t101 = t22+t45;
t148 = t33+t34+t40;
t67 = -t38;
t72 = t2.*t47;
t84 = -t44;
t97 = -t75;
t98 = -t76;
t99 = -t87;
t100 = -t89;
t102 = t20+t51;
t103 = t21+t50;
t104 = -t94;
t105 = -t95;
t111 = t11.*t101;
t115 = t42+t74;
t119 = t47+t71;
t155 = t36+t49+t96;
t157 = t43+t68+t73;
t106 = B_con_H.*t102;
t107 = B_con_H.*t103;
t108 = t19+t67;
t109 = t23+t84;
t110 = t3.*t102;
t112 = t9.*t102;
t113 = t9.*t103;
t114 = t13.*t103;
t120 = t15.*t102;
t121 = t15.*t103;
t122 = t16.*t102;
t123 = t16.*t103;
t125 = t3.*t7.*t103;
t129 = -t111;
t133 = T_fur_gap.*t115;
t134 = T_fur_gap.*t119;
t135 = int_point_tail.*t115;
t136 = int_point_tail.*t119;
t156 = t46+t66+t72;
t159 = T_fur_gap.*t155;
t161 = T_fur_gap.*t157;
t162 = int_point_tail.*t155;
t164 = int_point_tail.*t157;
t167 = t5.*t157;
t174 = t77+t78+t104;
t175 = t81+t82+t105;
t180 = t115.*t148;
t181 = t119.*t148;
t189 = t148.*t155;
t191 = t148.*t157;
t116 = B_con_H.*t108;
t117 = B_con_H.*t109;
t118 = -t107;
t124 = t7.*t110;
t126 = t3.*t114;
t127 = t7.*t113;
t128 = t3.*t108;
t130 = t9.*t108;
t131 = t9.*t109;
t132 = t13.*t109;
t137 = t15.*t108;
t138 = t15.*t109;
t139 = -t121;
t140 = t16.*t108;
t141 = t16.*t109;
t142 = -t123;
t144 = t3.*t7.*t109;
t154 = t85+t114;
t160 = T_fur_gap.*t156;
t163 = int_point_tail.*t156;
t166 = -t11.*(t48-t114);
t176 = T_fur_gap.*t174;
t177 = int_point_tail.*t174;
t178 = T_fur_gap.*t175;
t179 = int_point_tail.*t175;
t190 = t148.*t156;
t195 = t129+t167;
t210 = t148.*t174;
t212 = t148.*t175;
t220 = t134+t136+t181;
t223 = t161+t164+t191;
t224 = t65+t90+t93+t133+t135+t180;
t227 = t18+t24+t31+t56+t91+t159+t162+t189;
t143 = t7.*t128;
t145 = -t124;
t146 = t3.*t132;
t147 = t7.*t131;
t149 = -t128;
t150 = -t137;
t151 = -t138;
t158 = t41+t132;
t169 = t98+t126;
t171 = -T_fur_gap.*(t76-t126);
t173 = -int_point_tail.*(t76-t126);
t185 = -T_fur_gap.*(t124-t131);
t187 = -int_point_tail.*(t124-t131);
t188 = t79+t125+t130;
t194 = t97+t112+t144;
t207 = -t148.*(t76-t126);
t214 = -t148.*(t124-t131);
t228 = t17+t26+t63+t64+t92+t160+t163+t190;
t229 = t32+t55+t62+t88+t100+t178+t179+t212;
t230 = t29+t52+t57+t86+t99+t176+t177+t210;
t152 = -t143;
t153 = -t147;
t165 = t11.*t158;
t168 = t70+t146;
t183 = t131+t145;
t192 = T_fur_gap.*t188;
t193 = int_point_tail.*t188;
t197 = t83+t127+t149;
t198 = T_fur_gap.*t194;
t200 = int_point_tail.*t194;
t215 = t148.*t188;
t216 = t148.*t194;
t226 = t171+t173+t207;
t233 = t106+t122+t151+t185+t187+t214;
t170 = T_fur_gap.*t168;
t172 = int_point_tail.*t168;
t182 = t113+t152;
t196 = t80+t110+t153;
t201 = T_fur_gap.*t197;
t203 = int_point_tail.*t197;
t205 = t148.*t168;
t206 = t5.*t197;
t208 = -t198;
t209 = -t200;
t218 = t148.*t197;
t219 = -t216;
t235 = t30+t58+t118+t142+t150+t192+t193+t215;
t184 = T_fur_gap.*t182;
t186 = int_point_tail.*t182;
t199 = T_fur_gap.*t196;
t202 = int_point_tail.*t196;
t204 = t5.*t196;
t211 = -t206;
t213 = t148.*t182;
t217 = t148.*t196;
t225 = t170+t172+t205;
t232 = t201+t203+t218;
t236 = t25+t53+t117+t120+t141+t208+t209+t219;
t221 = t165+t204;
t222 = t166+t211;
t231 = t199+t202+t217;
t234 = t116+t139+t140+t184+t186+t213;
et1 = dphi1.*(t234.*(t206+t11.*(t48-t114))+(t111-t167).*(t28+t54+t61-t133-t135-t180)+t221.*(-t106-t122+t138+T_fur_gap.*(t124-t131)+int_point_tail.*(t124-t131)+t148.*(t124-t131))-t227.*(t5.*(t7.*t49-t2.*t3.*t6)-t6.*t8.*t11.*t13)+t236.*(t5.*(t3.*t109+t7.*t112)-t11.*t13.*t102)-t235.*(t5.*(t3.*t103+t7.*t130)-t11.*t13.*t108))+dphi2.*(t232.*(t206+t11.*(t48-t114))+t221.*t231-t223.*(t111-t167)-t5.*t155.*t227-t5.*t188.*t235+t5.*t194.*t236);
et2 = dth1.*(t229.*(t206+t11.*(t48-t114))+t221.*t230-t228.*(t111-t167)-t227.*(t11.*(t6.*t7-t2.*t12.*t13)+t5.*(t3.*t8.*t12+t6.*t9.*t13+t2.*t9.*t22))+t236.*(t11.*(t4.*t22+t6.*t13.*t19)-t5.*(t4.*t68+t3.*t6.*t21+t6.*t7.*t9.*t19))+t235.*(t11.*(t10.*t22+t6.*t13.*t20)-t5.*(t10.*t68+t3.*t6.*t23+t6.*t7.*t9.*t20)))+dy.*(t108.*(t206+t11.*(t48-t114))-t102.*t221+t6.*t8.*(t111-t167))-dz.*(-t103.*(t206+t11.*(t48-t114))+t109.*t221+t2.*t6.*(t111-t167));
et3 = -dth2.*(-t227.*(t11.*(t12.*t13-t2.*t6.*t7)-t5.*(t9.*t22+t13.*t42))-t235.*(t11.*(t7.*t103+t6.*t10.*t13)-t5.*(t9.*t48-t13.*t113))+t236.*(t11.*(t7.*t109-t4.*t6.*t13)+t5.*(t9.*t41+t13.*t131))+t221.*t225+(t206+t11.*(t48-t114)).*(T_fur_gap.*(t76-t126)+int_point_tail.*(t76-t126)+t148.*(t76-t126))+t220.*(t111-t167))-dx.*(t12.*(t111-t167)+t6.*t10.*(t206+t11.*(t48-t114))+t4.*t6.*t221)+t5.*windspeed.*(t206+t11.*(t48-t114))+t11.*t221.*windspeed;
et4 = -dphi1.*(t155.*(t28+t54+t61-t133-t135-t180)-t115.*t227+t182.*t235+t188.*t234+t236.*(t124-t131)-t194.*(-t106-t122+t138+T_fur_gap.*(t124-t131)+int_point_tail.*(t124-t131)+t148.*(t124-t131)))+dth2.*(t119.*t227+t155.*t220+t168.*t236-t194.*t225+t188.*(T_fur_gap.*(t76-t126)+int_point_tail.*(t76-t126)+t148.*(t76-t126))+t235.*(t76-t126))-dy.*(t102.*t194+t108.*t188+t6.*t8.*t155)-dz.*(t103.*t188+t109.*t194-t2.*t6.*t155)+dphi2.*(t155.*t223+t157.*t227-t188.*t232+t194.*t231-t196.*t236-t197.*t235);
et5 = dth1.*(t155.*t228+t156.*t227-t174.*t236-t175.*t235-t188.*t229+t194.*t230)+dx.*(t12.*t155-t4.*t6.*t194+t6.*t10.*t188)-t5.*t188.*windspeed+t11.*t194.*windspeed;
aoa_tail_2 = th2-atan((et4+et5)./(et1+et2+et3));

== matlab function SimulinkAnalysisofCheetahTail/Model/Forces/CD_CL_tail_3/v_tail_3 ==
  data: int_point_tail input; q input; dq input; v_tail_3_speed output; psi3 parameter; windspeed parameter; B_con_H parameter; B_con_L parameter; M_cg_H parameter; M_cg_L parameter; M_cg_W parameter; T_fur_gap parameter; T_length parameter; bar_len parameter
function v_tail_3_speed = v_tail_3(int_point_tail,q,dq, psi3, windspeed, B_con_H, B_con_L, M_cg_H, M_cg_L, M_cg_W, T_fur_gap, T_length, bar_len)
%#codegen
[x,y,z,phi1,th1,psi1,phi2,th2] = deal(q(1),q(2),q(3),q(4),q(5),q(6),q(7),q(8));
[dx,dy,dz,dphi1,dth1,dpsi1,dphi2,dth2] = deal(dq(1),dq(2),dq(3),dq(4),dq(5),dq(6),dq(7),dq(8));
%    This function was generated by the Symbolic Math Toolbox version 9.0.
%    09-Feb-2022 11:07:26

t2 = cos(phi1);
t3 = cos(phi2);
t4 = cos(psi1);
t5 = cos(psi3);
t6 = cos(th1);
t7 = cos(th2);
t8 = sin(phi1);
t9 = sin(phi2);
t10 = sin(psi1);
t11 = sin(psi3);
t12 = sin(th1);
t13 = sin(th2);
t14 = M_cg_L+x;
t15 = M_cg_W+y;
t16 = M_cg_H+z;
t26 = T_length./2.0;
t27 = bar_len./2.0;
t28 = int_point_tail./2.0;
t17 = B_con_L.*t6;
t18 = B_con_L.*t12;
t19 = t2.*t4;
t20 = t6.*t7;
t21 = t2.*t10;
t22 = t4.*t8;
t23 = t7.*t12;
t24 = t8.*t10;
t25 = t12.*t13;
t29 = B_con_H.*t2.*t6;
t31 = t6.*t14;
t32 = B_con_H.*t2.*t12;
t33 = B_con_H.*t6.*t8;
t36 = t12.*t14;
t38 = -t28;
t41 = t6.*t9.*t13;
t43 = t6.*t10.*t13;
t45 = t8.*t9.*t12;
t48 = t2.*t3.*t6;
t51 = t2.*t6.*t9;
t52 = t3.*t6.*t8;
t54 = t2.*t6.*t13;
t55 = t3.*t6.*t13;
t57 = t4.*t6.*t13;
t60 = t3.*t8.*t12;
t61 = t6.*t8.*t9;
t66 = t2.*t6.*t15;
t68 = t2.*t6.*t16;
t71 = t6.*t8.*t15;
t72 = t2.*t12.*t16;
t73 = t6.*t8.*t16;
t75 = t8.*t12.*t15;
t30 = t4.*t17;
t34 = t4.*t18;
t35 = t10.*t17;
t37 = t10.*t18;
t39 = t2.*t25;
t40 = t3.*t25;
t42 = t9.*t23;
t44 = t10.*t23;
t46 = t12.*t24;
t47 = t9.*t25;
t49 = t2.*t20;
t50 = t4.*t20;
t53 = t12.*t19;
t56 = t3.*t23;
t58 = t4.*t23;
t59 = t10.*t20;
t62 = t12.*t21;
t63 = t12.*t22;
t64 = B_con_H.*t6.*t19;
t65 = t4.*t31;
t67 = B_con_H.*t6.*t21;
t69 = t4.*t36;
t70 = t10.*t31;
t74 = t10.*t36;
t76 = -t32;
t77 = -t33;
t79 = -t45;
t84 = t3.*t6.*t22;
t85 = t13.*t48;
t88 = t3.*t8.*t20;
t89 = t6.*t13.*t19;
t90 = t4.*t55;
t93 = t3.*t6.*t24;
t94 = t6.*t9.*t22;
t95 = t2.*t41;
t97 = t8.*t9.*t20;
t98 = t6.*t13.*t21;
t100 = t3.*t43;
t101 = t4.*t41;
t103 = t6.*t9.*t24;
t107 = t10.*t41;
t109 = -t57;
t112 = t6.*t16.*t19;
t113 = t6.*t15.*t22;
t114 = t6.*t16.*t21;
t115 = t6.*t15.*t24;
t116 = -t66;
t117 = -t71;
t118 = -t72;
t119 = -t73;
t120 = t3.*t19.*t20;
t121 = t3.*t20.*t21;
t122 = t9.*t19.*t20;
t123 = t9.*t20.*t21;
t133 = t23+t54;
t160 = t26+t27+t38;
t78 = -t39;
t80 = -t46;
t81 = -t47;
t82 = t3.*t49;
t83 = t3.*t50;
t86 = t2.*t56;
t87 = t9.*t49;
t91 = t3.*t59;
t92 = t9.*t50;
t96 = t2.*t42;
t99 = t4.*t40;
t102 = t9.*t59;
t104 = -t49;
t105 = t10.*t40;
t106 = t4.*t47;
t108 = -t53;
t110 = -t59;
t111 = t10.*t47;
t125 = -t90;
t127 = -t97;
t131 = -t113;
t132 = -t115;
t134 = t21+t63;
t135 = t22+t62;
t136 = -t120;
t137 = -t121;
t144 = t5.*t133;
t148 = t11.*t133;
t152 = t51+t88;
t156 = t56+t85;
t157 = t58+t89;
t158 = t42+t95;
t159 = t44+t98;
t124 = -t82;
t126 = -t91;
t128 = -t102;
t129 = t4.*t81;
t130 = t10.*t81;
t138 = B_con_H.*t134;
t139 = B_con_H.*t135;
t140 = t20+t78;
t141 = t25+t104;
t142 = t19+t80;
t143 = t24+t108;
t145 = t3.*t134;
t146 = t3.*t135;
t147 = t7.*t135;
t149 = t9.*t134;
t150 = t9.*t135;
t151 = t13.*t135;
t161 = t15.*t134;
t162 = t15.*t135;
t163 = t16.*t134;
t164 = t16.*t135;
t174 = -t148;
t178 = t48+t127;
t179 = T_fur_gap.*t152;
t180 = T_fur_gap.*t156;
t181 = int_point_tail.*t152;
t182 = int_point_tail.*t156;
t202 = t41+t60+t96;
t205 = t55+t79+t86;
t206 = t52+t81+t87;
t229 = t94+t99+t136;
t231 = t103+t105+t137;
t237 = t152.*t160;
t238 = t156.*t160;
t153 = B_con_H.*t142;
t154 = B_con_H.*t143;
t155 = -t139;
t165 = t7.*t145;
t166 = t7.*t146;
t167 = t13.*t146;
t168 = t7.*t149;
t169 = t9.*t147;
t170 = t13.*t150;
t171 = t3.*t142;
t172 = t3.*t143;
t173 = t7.*t143;
t175 = t9.*t142;
t176 = t9.*t143;
t177 = t13.*t143;
t183 = t15.*t142;
t184 = t15.*t143;
t185 = -t162;
t186 = t16.*t142;
t187 = t16.*t143;
t188 = -t164;
t201 = t43+t147;
t203 = t110+t151;
t204 = t40+t61+t124;
t209 = T_fur_gap.*t205;
t210 = T_fur_gap.*t206;
t212 = int_point_tail.*t205;
t213 = int_point_tail.*t206;
t216 = -t5.*(t59-t151);
t218 = -t11.*(t59-t151);
t219 = t5.*t206;
t220 = t11.*t206;
t230 = t84+t122+t129;
t232 = t93+t123+t130;
t233 = T_fur_gap.*t229;
t234 = int_point_tail.*t229;
t235 = T_fur_gap.*t231;
t236 = int_point_tail.*t231;
t248 = t160.*t205;
t249 = t160.*t206;
t266 = t160.*t229;
t267 = t160.*t231;
t283 = t180+t182+t238;
t289 = t77+t116+t119+t179+t181+t237;
t189 = t7.*t171;
t190 = t7.*t172;
t191 = -t165;
t192 = t13.*t172;
t193 = t7.*t175;
t194 = t9.*t173;
t195 = t13.*t176;
t196 = -t171;
t197 = -t183;
t198 = -t184;
t207 = t50+t177;
t208 = T_fur_gap.*t204;
t211 = int_point_tail.*t204;
t214 = t109+t173;
t222 = t126+t167;
t224 = t128+t170;
t226 = -T_fur_gap.*(t91-t167);
t228 = -int_point_tail.*(t91-t167);
t240 = t168+t172;
t244 = -T_fur_gap.*(t165-t176);
t246 = -int_point_tail.*(t165-t176);
t247 = t160.*t204;
t250 = t144+t220;
t251 = t100+t166+t175;
t255 = t174+t219;
t259 = -t160.*(t91-t167);
t277 = -t160.*(t165-t176);
t288 = t210+t213+t249;
t293 = t17+t31+t75+t76+t118+t209+t212+t248;
t294 = t37+t67+t74+t114+t132+t235+t236+t267;
t295 = t34+t64+t69+t112+t131+t233+t234+t266;
t199 = -t189;
t200 = -t194;
t215 = t5.*t207;
t217 = t11.*t207;
t221 = t83+t192;
t223 = t92+t195;
t239 = t146+t193;
t242 = t176+t191;
t252 = T_fur_gap.*t251;
t253 = int_point_tail.*t251;
t254 = t125+t149+t190;
t257 = t107+t169+t196;
t278 = t160.*t251;
t291 = t226+t228+t259;
t292 = t18+t29+t36+t68+t117+t208+t211+t247;
t298 = t138+t163+t198+t244+t246+t277;
t225 = T_fur_gap.*t221;
t227 = int_point_tail.*t221;
t241 = t150+t199;
t256 = t101+t145+t200;
t258 = t160.*t221;
t260 = T_fur_gap.*t254;
t262 = int_point_tail.*t254;
t263 = T_fur_gap.*t257;
t265 = int_point_tail.*t257;
t269 = t5.*t257;
t271 = t11.*t257;
t279 = t160.*t254;
t281 = t160.*t257;
t300 = t35+t70+t155+t188+t197+t252+t253+t278;
t243 = T_fur_gap.*t241;
t245 = int_point_tail.*t241;
t261 = T_fur_gap.*t256;
t264 = int_point_tail.*t256;
t268 = t5.*t256;
t270 = t11.*t256;
t272 = -t260;
t273 = -t262;
t274 = -t269;
t276 = t160.*t241;
t280 = t160.*t256;
t282 = -t279;
t285 = t216+t271;
t290 = t225+t227+t258;
t297 = t263+t265+t281;
t275 = -t270;
t284 = t217+t268;
t287 = t218+t274;
t296 = t261+t264+t280;
t299 = t153+t185+t186+t243+t245+t276;
t301 = t30+t65+t154+t161+t187+t272+t273+t282;
t286 = t215+t275;
et1 = dphi1.*(t204.*(t33+t66+t73-t179-t181-t237)-t152.*t292+t241.*t300+t251.*t299+t301.*(t165-t176)-t254.*(-t138-t163+t184+T_fur_gap.*(t165-t176)+int_point_tail.*(t165-t176)+t160.*(t165-t176)))-dth2.*(t156.*t292+t204.*t283+t221.*t301-t254.*t290+t251.*(T_fur_gap.*(t91-t167)+int_point_tail.*(t91-t167)+t160.*(t91-t167))+t300.*(t91-t167))+dy.*(t134.*t254+t142.*t251+t6.*t8.*t204)+dz.*(t135.*t251+t143.*t254-t2.*t6.*t204)-dphi2.*(t204.*t288+t206.*t292-t251.*t297+t254.*t296-t256.*t301-t257.*t300);
et2 = -dth1.*(t204.*t293+t205.*t292-t229.*t301-t231.*t300-t251.*t294+t254.*t295)-dx.*(t12.*t204-t4.*t6.*t254+t6.*t10.*t251)+t5.*t251.*windspeed-t11.*t254.*windspeed;
et3 = dphi2.*(t297.*(t271-t5.*(t59-t151))+t250.*t288-t286.*t296-t11.*t204.*t292-t11.*t251.*t300+t11.*t254.*t301)+dth1.*(t294.*(t271-t5.*(t59-t151))+t250.*t293-t286.*t295+t292.*(t5.*t140-t11.*t202)-t301.*(t5.*t157+t11.*t230)-t300.*(t5.*t159+t11.*t232))+dy.*(t142.*(t271-t5.*(t59-t151))+t134.*t286-t6.*t8.*t250)+dz.*(t135.*(t271-t5.*(t59-t151))+t143.*t286+t2.*t6.*t250);
et4 = -dth2.*(-t250.*t283-t286.*t290+(t271-t5.*(t59-t151)).*(T_fur_gap.*(t91-t167)+int_point_tail.*(t91-t167)+t160.*(t91-t167))+t292.*(t5.*t141+t11.*t158)+t301.*(t11.*t223+t5.*(t57-t173))+t300.*(t5.*t201+t11.*(t102-t170)))+dx.*(t12.*t250-t6.*t10.*(t271-t5.*(t59-t151))+t4.*t6.*t286);
et5 = -dphi1.*(t250.*(t33+t66+t73-t179-t181-t237)-t299.*(t271-t5.*(t59-t151))-t301.*(t11.*t240+t5.*t13.*t134)+t300.*(t11.*t239+t5.*t13.*t142)+t286.*(-t138-t163+t184+T_fur_gap.*(t165-t176)+int_point_tail.*(t165-t176)+t160.*(t165-t176))-t292.*(t11.*t178-t5.*t6.*t8.*t13))+t5.*windspeed.*(t271-t5.*(t59-t151))-t11.*t286.*windspeed;
et6 = -dphi1.*(t299.*(t269+t11.*(t59-t151))+t301.*(t5.*t240-t11.*t13.*t134)-t300.*(t5.*t239-t11.*t13.*t142)+(t148-t219).*(t33+t66+t73-t179-t181-t237)+t284.*(-t138-t163+t184+T_fur_gap.*(t165-t176)+int_point_tail.*(t165-t176)+t160.*(t165-t176))+t292.*(t5.*t178+t6.*t8.*t11.*t13))-dphi2.*(t297.*(t269+t11.*(t59-t151))+t284.*t296-t288.*(t148-t219)-t5.*t204.*t292-t5.*t251.*t300+t5.*t254.*t301);
et7 = -dth1.*(t294.*(t269+t11.*(t59-t151))+t284.*t295-t293.*(t148-t219)-t292.*(t11.*t140+t5.*t202)+t301.*(t11.*t157-t5.*t230)+t300.*(t11.*t159-t5.*t232))-dy.*(t142.*(t269+t11.*(t59-t151))-t134.*t284+t6.*t8.*(t148-t219))+dz.*(-t135.*(t269+t11.*(t59-t151))+t143.*t284+t2.*t6.*(t148-t219));
et8 = dth2.*(t284.*t290+(t269+t11.*(t59-t151)).*(T_fur_gap.*(t91-t167)+int_point_tail.*(t91-t167)+t160.*(t91-t167))+t283.*(t148-t219)-t292.*(t11.*t141-t5.*t158)+t301.*(t5.*t223-t11.*(t57-t173))-t300.*(t11.*t201-t5.*(t102-t170)))+dx.*(t12.*(t148-t219)+t6.*t10.*(t269+t11.*(t59-t151))+t4.*t6.*t284)-t5.*windspeed.*(t269+t11.*(t59-t151))-t11.*t284.*windspeed;
v_tail_3_speed = sqrt(abs(et3+et4+et5).^2+abs(et6+et7+et8).^2+abs(et1+et2).^2);
